simulink model "platoon_blocks_hills"  (R2015b)
settings: Solver=VariableStepAuto  StartTime=0.0  StopTime=50.0  MaxStep=0.001  RelTol=1e-3
undefined symbols (not defined in the file or in its folder): ca1_2, ca1_3, ca1_4, ca1_5, ca1_6, caf1_3, caf1_4, caf1_5, caf1_6, cv1_2, cv1_3, cv1_4, cv1_5, cv1_6, cvf1_3, cvf1_4, cvf1_5, cvf1_6, cx1_2, cx1_3, cx1_4, cx1_5, cx1_6, theta_hill, x_hill
settings Model: Creator=cf5eg  LastModifiedBy=cf5eg

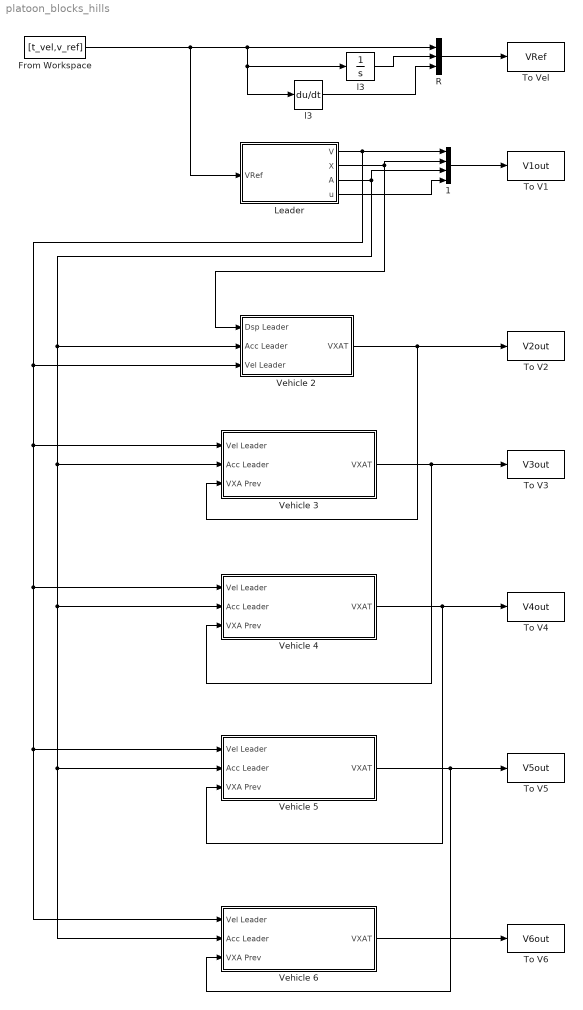
== system platoon_blocks_hills ==
  " 1" : Concatenate  NumInputs=4
  " R" : Concatenate  NumInputs=3
  " l3" : Derivative
  From Workspace : FromWorkspace  VariableName=[t_vel,v_ref]  SampleTime=0
  Leader : Subsystem
  To V1 : ToWorkspace  VariableName=V1out  SaveFormat=Timeseries  SampleTime=-1
  To V2 : ToWorkspace  VariableName=V2out  SaveFormat=Timeseries  SampleTime=-1
  To V3 : ToWorkspace  VariableName=V3out  SaveFormat=Timeseries  SampleTime=-1
  To V4 : ToWorkspace  VariableName=V4out  SaveFormat=Timeseries  SampleTime=-1
  To V5 : ToWorkspace  VariableName=V5out  SaveFormat=Timeseries  SampleTime=-1
  To V6 : ToWorkspace  VariableName=V6out  SaveFormat=Timeseries  SampleTime=-1
  To Vel : ToWorkspace  VariableName=VRef  SaveFormat=Timeseries  SampleTime=-1
  Vehicle 2 : Subsystem
  Vehicle 3 : Subsystem
  Vehicle 4 : Subsystem
  Vehicle 5 : Subsystem
      mask Display: image('car.jpg')
  Vehicle 6 : Subsystem
      mask Display: image('car.jpg')
  l3 : Integrator
  wires:
  " 1"/1 -> To V1/1
  Vehicle 3/1(VXAT) -> Vehicle 4/3(VXA Prev), To V3/1
  l3/1 -> " R"/2
  " l3"/1 -> " R"/3
  " R"/1 -> To Vel/1
  From Workspace/1 -> Leader/1(VRef), " l3"/1, l3/1, " R"/1
  Vehicle 4/1(VXAT) -> Vehicle 5/3(VXA Prev), To V4/1
  Vehicle 5/1(VXAT) -> Vehicle 6/3(VXA Prev), To V5/1
  Leader/2(X) -> Vehicle 2/1(Dsp Leader), " 1"/2
  Leader/3(A) -> " 1"/3, Vehicle 2/2(Acc Leader), Vehicle 6/2(Acc Leader), Vehicle 5/2(Acc Leader), Vehicle 4/2(Acc Leader), Vehicle 3/2(Acc Leader)
  Leader/1(V) -> " 1"/1, Vehicle 2/3(Vel Leader), Vehicle 6/1(Vel Leader), Vehicle 5/1(Vel Leader), Vehicle 4/1(Vel Leader), Vehicle 3/1(Vel Leader)
  Vehicle 6/1(VXAT) -> To V6/1
  Vehicle 2/1(VXAT) -> Vehicle 3/3(VXA Prev), To V2/1
  Leader/4(u) -> " 1"/4

== system platoon_blocks_hills/Leader ==
  VRef : Inport
  " l" : Derivative
  Der Error : Derivative
  Int Error : Integrator
  Sum5 : Sum  Inputs=+++
  Sum7 : Sum  Inputs=|+-
  Transport Delay : TransportDelay  DelayTime=0.1
  Vehicle 1 : Subsystem
  kd : Gain  Gain=0
  ki : Gain  Gain=0.1
  kp : Gain  Gain=0.5
  l : Integrator
  V : Outport
  X : Outport  Port=2
  A : Outport  Port=3
  u : Outport  Port=4
  wires:
  VRef/1 -> Sum7/1
  Sum5/1 -> Transport Delay/1
  Vehicle 1/1(v) -> l/1, Sum7/2, " l"/1, V/1
  Sum7/1 -> Der Error/1, Int Error/1, kp/1
  kp/1 -> Sum5/1
  ki/1 -> Sum5/2
  Int Error/1 -> ki/1
  kd/1 -> Sum5/3
  Der Error/1 -> kd/1
  l/1 -> X/1
  " l"/1 -> A/1
  Transport Delay/1 -> Vehicle 1/1(u)
  Vehicle 1/2(throttle) -> u/1

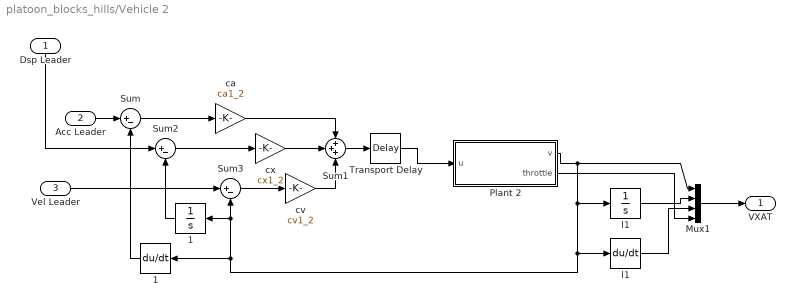
== system platoon_blocks_hills/Vehicle 2 ==
  Dsp Leader : Inport
  Acc Leader : Inport  Port=2
  Vel Leader : Inport  Port=3
  " l1" : Derivative
  1 : Integrator
  "1 " : Derivative
  Mux1 : Mux
  Plant 2 : Subsystem
  Sum : Sum  Inputs=|+-
  Sum1 : Sum  Inputs=+++
  Sum2 : Sum  Inputs=|+-
  Sum3 : Sum  Inputs=|+-
  Transport Delay : TransportDelay  DelayTime=0.1
  ca : Gain  Gain=ca1_2
  cv : Gain  Gain=cv1_2
  cx : Gain  Gain=cx1_2
  l1 : Integrator
  VXAT : Outport
  wires:
  Vel Leader/1 -> Sum3/1
  ca/1 -> Sum1/1
  Sum2/1 -> cx/1
  cx/1 -> Sum1/2
  cv/1 -> Sum1/3
  Sum/1 -> ca/1
  1/1 -> Sum2/2
  "1 "/1 -> Sum/2
  Sum3/1 -> cv/1
  Sum1/1 -> Transport Delay/1
  Plant 2/1(v) -> Mux1/1, l1/1, " l1"/1, Sum3/2, 1/1, "1 "/1
  " l1"/1 -> Mux1/3
  l1/1 -> Mux1/2
  Dsp Leader/1 -> Sum2/1
  Acc Leader/1 -> Sum/1
  Mux1/1 -> VXAT/1
  Transport Delay/1 -> Plant 2/1(u)
  Plant 2/2(throttle) -> Mux1/4

== system platoon_blocks_hills/Vehicle 3 ==
  Vel Leader : Inport
  Acc Leader : Inport  Port=2
  VXA Prev : Inport  Port=3
  Controller 3 : Subsystem
  Demux : Demux
  Mux1 : Mux
  Plant 3 : Subsystem
  Terminator : Terminator
  Transport Delay : TransportDelay  DelayTime=0.1
  VXAT : Outport
  wires:
  Controller 3/1(u) -> Transport Delay/1
  Plant 3/1(v) -> Mux1/1, Controller 3/6(vself)
  Plant 3/2(x) -> Mux1/2
  Plant 3/3(a) -> Mux1/3
  Vel Leader/1 -> Controller 3/2(vl)
  Acc Leader/1 -> Controller 3/1(al)
  VXA Prev/1 -> Demux/1
  Demux/1 -> Controller 3/5(v0)
  Demux/2 -> Controller 3/4(x0)
  Demux/3 -> Controller 3/3(a0)
  Mux1/1 -> VXAT/1
  Transport Delay/1 -> Plant 3/1(u)
  Demux/4 -> Terminator/1
  Plant 3/4(t) -> Mux1/4

== system platoon_blocks_hills/Vehicle 4 ==
  Vel Leader : Inport
  Acc Leader : Inport  Port=2
  VXA Prev : Inport  Port=3
  Controller 4 : Subsystem
  Demux : Demux
  Mux1 : Mux
  Plant 4 : Subsystem
  Terminator : Terminator
  Transport Delay : TransportDelay  DelayTime=0.1
  VXAT : Outport
  wires:
  Controller 4/1(u) -> Transport Delay/1
  Plant 4/1(v) -> Controller 4/6(vself), Mux1/1
  Plant 4/2(x) -> Mux1/2
  Plant 4/3(a) -> Mux1/3
  Vel Leader/1 -> Controller 4/2(vl)
  Acc Leader/1 -> Controller 4/1(al)
  VXA Prev/1 -> Demux/1
  Demux/1 -> Controller 4/5(v0)
  Demux/2 -> Controller 4/4(x0)
  Demux/3 -> Controller 4/3(a0)
  Mux1/1 -> VXAT/1
  Transport Delay/1 -> Plant 4/1(u)
  Demux/4 -> Terminator/1
  Plant 4/4(t) -> Mux1/4

== system platoon_blocks_hills/Vehicle 5 ==
  Vel Leader : Inport
  Acc Leader : Inport  Port=2
  VXA Prev : Inport  Port=3
  Controller 5 : Subsystem
  Demux : Demux
  Mux1 : Mux
  Plant 5 : Subsystem
  Terminator : Terminator
  Transport Delay : TransportDelay  DelayTime=0.1
  VXAT : Outport
  wires:
  Controller 5/1(u) -> Transport Delay/1
  Plant 5/1(v) -> Controller 5/6(vself), Mux1/1
  Plant 5/2(x) -> Mux1/2
  Plant 5/3(a) -> Mux1/3
  Vel Leader/1 -> Controller 5/2(vl)
  Acc Leader/1 -> Controller 5/1(al)
  VXA Prev/1 -> Demux/1
  Demux/1 -> Controller 5/5(v0)
  Demux/2 -> Controller 5/4(x0)
  Demux/3 -> Controller 5/3(a0)
  Mux1/1 -> VXAT/1
  Transport Delay/1 -> Plant 5/1(u)
  Demux/4 -> Terminator/1
  Plant 5/4(t) -> Mux1/4

== system platoon_blocks_hills/Vehicle 6 ==
  Vel Leader : Inport
  Acc Leader : Inport  Port=2
  VXA Prev : Inport  Port=3
  Controller 6 : Subsystem
  Demux : Demux
  Mux1 : Mux
  Plant 6 : Subsystem
  Terminator : Terminator
  Transport Delay : TransportDelay  DelayTime=0.1
  VXAT : Outport
  wires:
  Controller 6/1(u) -> Transport Delay/1
  Plant 6/1(v) -> Controller 6/6(vself), Mux1/1
  Plant 6/2(x) -> Mux1/2
  Plant 6/3(a) -> Mux1/3
  Acc Leader/1 -> Controller 6/1(al)
  VXA Prev/1 -> Demux/1
  Mux1/1 -> VXAT/1
  Transport Delay/1 -> Plant 6/1(u)
  Demux/3 -> Controller 6/3(a0)
  Demux/2 -> Controller 6/4(x0)
  Demux/1 -> Controller 6/5(v0)
  Vel Leader/1 -> Controller 6/2(vl)
  Demux/4 -> Terminator/1
  Plant 6/4(t) -> Mux1/4

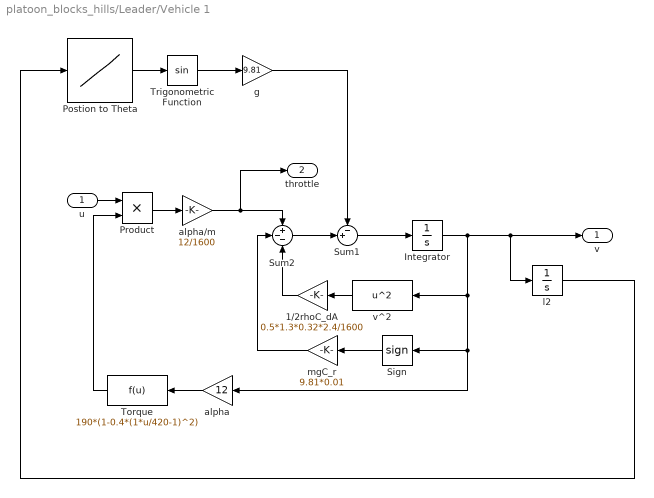
== system platoon_blocks_hills/Leader/Vehicle 1 ==
  u : Inport
  1/2rhoC_dA : Gain  Gain=0.5*1.3*0.32*2.4/1600
  Integrator : Integrator
  Postion to Theta : Lookup_n-D  NumberOfTableDimensions=1  BreakpointsForDimension1=x_hill  Table=theta_hill  InternalRulePriority=Speed  RndMeth=Simplest  InputSameDT=on
  Product : Product
  Sign : Signum  ZeroCross=off
  Sum1 : Sum  Inputs=-+|
  Sum2 : Sum  Inputs=+--
  Torque : Fcn  Expr=190*(1-0.4*(1*u/420-1)^2)
  Trigonometric Function : Trigonometry
  alpha : Gain  Gain=12
  alpha/m : Gain  Gain=12/1600
  g : Gain  Gain=9.81
  l2 : Integrator
  "mgC_r " : Gain  Gain=9.81*0.01
  v^2 : Fcn  Expr=u^2
  v : Outport
  throttle : Outport  Port=2
  wires:
  Product/1 -> alpha/m/1
  alpha/m/1 -> throttle/1, Sum2/1
  alpha/1 -> Torque/1
  Torque/1 -> Product/2
  v^2/1 -> 1/2rhoC_dA/1
  1/2rhoC_dA/1 -> Sum2/3
  Integrator/1 -> l2/1, v/1, Sign/1, alpha/1, v^2/1
  Sum2/1 -> Sum1/2
  "mgC_r "/1 -> Sum2/2
  Sign/1 -> "mgC_r "/1
  u/1 -> Product/1
  l2/1 -> Postion to Theta/1
  Postion to Theta/1 -> Trigonometric Function/1
  Trigonometric Function/1 -> g/1
  Sum1/1 -> Integrator/1
  g/1 -> Sum1/1

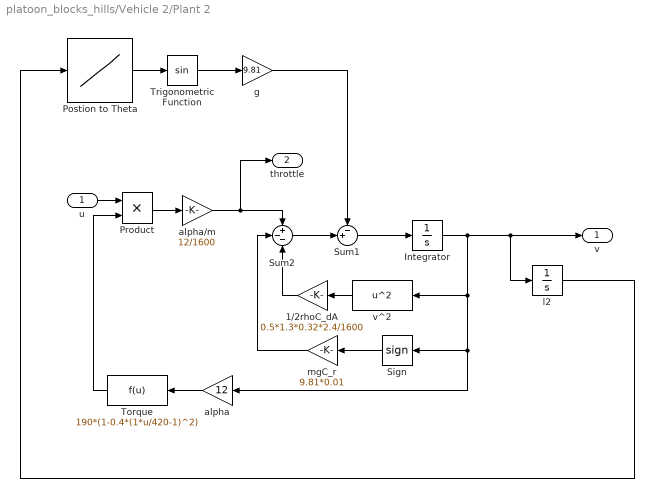
== system platoon_blocks_hills/Vehicle 2/Plant 2 ==
  u : Inport
  1/2rhoC_dA : Gain  Gain=0.5*1.3*0.32*2.4/1600
  Integrator : Integrator
  Postion to Theta : Lookup_n-D  NumberOfTableDimensions=1  BreakpointsForDimension1=x_hill  Table=theta_hill  InternalRulePriority=Speed  RndMeth=Simplest  InputSameDT=on
  Product : Product
  Sign : Signum  ZeroCross=off
  Sum1 : Sum  Inputs=-+|
  Sum2 : Sum  Inputs=+--
  Torque : Fcn  Expr=190*(1-0.4*(1*u/420-1)^2)
  Trigonometric Function : Trigonometry
  alpha : Gain  Gain=12
  alpha/m : Gain  Gain=12/1600
  g : Gain  Gain=9.81
  l2 : Integrator
  "mgC_r " : Gain  Gain=9.81*0.01
  v^2 : Fcn  Expr=u^2
  v : Outport
  throttle : Outport  Port=2
  wires:
  Product/1 -> alpha/m/1
  alpha/m/1 -> throttle/1, Sum2/1
  alpha/1 -> Torque/1
  Torque/1 -> Product/2
  v^2/1 -> 1/2rhoC_dA/1
  1/2rhoC_dA/1 -> Sum2/3
  Integrator/1 -> l2/1, v/1, Sign/1, alpha/1, v^2/1
  Sum2/1 -> Sum1/2
  "mgC_r "/1 -> Sum2/2
  Sign/1 -> "mgC_r "/1
  u/1 -> Product/1
  l2/1 -> Postion to Theta/1
  Postion to Theta/1 -> Trigonometric Function/1
  Trigonometric Function/1 -> g/1
  Sum1/1 -> Integrator/1
  g/1 -> Sum1/1

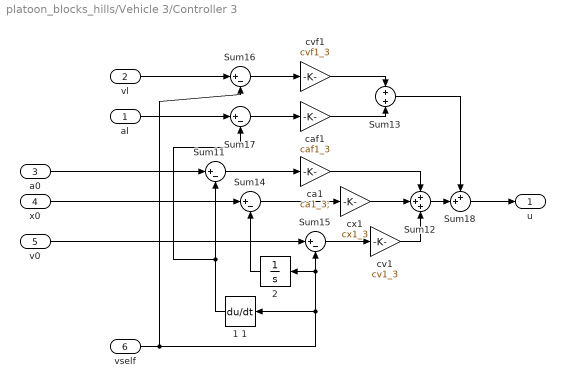
== system platoon_blocks_hills/Vehicle 3/Controller 3 ==
  al : Inport
  vl : Inport  Port=2
  a0 : Inport  Port=3
  x0 : Inport  Port=4
  v0 : Inport  Port=5
  vself : Inport  Port=6
  1 1 : Derivative
  2 : Integrator
  Sum{11,14..17} (5 alike) : Sum  Inputs=|+-
  Sum12 : Sum  Inputs=+++
  Sum13 : Sum  Inputs=+|+
  Sum18 : Sum  Inputs=++|
  ca1 : Gain  Gain=ca1_3;
  caf1 : Gain  Gain=caf1_3
  cv1 : Gain  Gain=cv1_3
  cvf1 : Gain  Gain=cvf1_3
  cx1 : Gain  Gain=cx1_3
  u : Outport
  wires:
  vl/1 -> Sum16/1
  ca1/1 -> Sum12/1
  Sum18/1 -> u/1
  Sum14/1 -> cx1/1
  cx1/1 -> Sum12/2
  cv1/1 -> Sum12/3
  Sum11/1 -> ca1/1
  2/1 -> Sum14/2
  1 1/1 -> Sum17/2, Sum11/2
  Sum15/1 -> cv1/1
  Sum16/1 -> cvf1/1
  Sum17/1 -> caf1/1
  caf1/1 -> Sum13/2
  cvf1/1 -> Sum13/1
  Sum12/1 -> Sum18/2
  Sum13/1 -> Sum18/1
  vself/1 -> Sum16/2, Sum15/2, 2/1, 1 1/1
  al/1 -> Sum17/1
  a0/1 -> Sum11/1
  v0/1 -> Sum15/1
  x0/1 -> Sum14/1

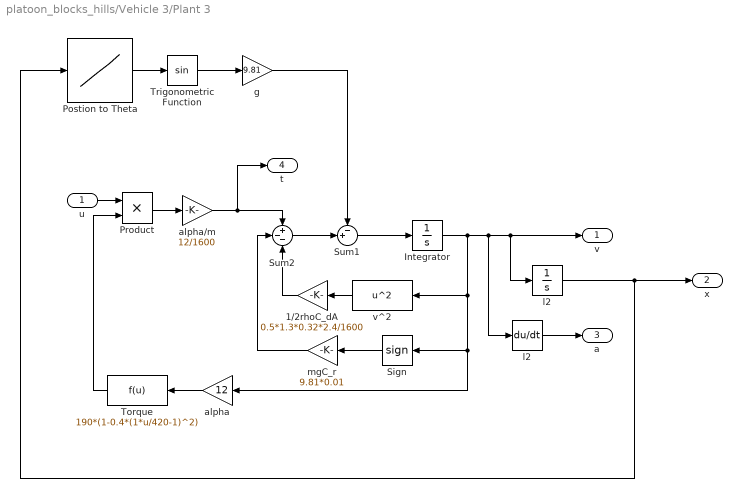
== system platoon_blocks_hills/Vehicle 3/Plant 3 ==
  u : Inport
  " l2" : Derivative
  1/2rhoC_dA : Gain  Gain=0.5*1.3*0.32*2.4/1600
  Integrator : Integrator
  Postion to Theta : Lookup_n-D  NumberOfTableDimensions=1  BreakpointsForDimension1=x_hill  Table=theta_hill  InternalRulePriority=Speed  RndMeth=Simplest  InputSameDT=on
  Product : Product
  Sign : Signum  ZeroCross=off
  Sum1 : Sum  Inputs=-+|
  Sum2 : Sum  Inputs=+--
  Torque : Fcn  Expr=190*(1-0.4*(1*u/420-1)^2)
  Trigonometric Function : Trigonometry
  alpha : Gain  Gain=12
  alpha/m : Gain  Gain=12/1600
  g : Gain  Gain=9.81
  l2 : Integrator
  "mgC_r " : Gain  Gain=9.81*0.01
  v^2 : Fcn  Expr=u^2
  v : Outport
  x : Outport  Port=2
  a : Outport  Port=3
  t : Outport  Port=4
  wires:
  Product/1 -> alpha/m/1
  alpha/m/1 -> t/1, Sum2/1
  alpha/1 -> Torque/1
  Torque/1 -> Product/2
  v^2/1 -> 1/2rhoC_dA/1
  1/2rhoC_dA/1 -> Sum2/3
  Integrator/1 -> " l2"/1, l2/1, v/1, Sign/1, alpha/1, v^2/1
  Sum2/1 -> Sum1/2
  "mgC_r "/1 -> Sum2/2
  Sign/1 -> "mgC_r "/1
  u/1 -> Product/1
  " l2"/1 -> a/1
  l2/1 -> x/1, Postion to Theta/1
  Postion to Theta/1 -> Trigonometric Function/1
  Trigonometric Function/1 -> g/1
  Sum1/1 -> Integrator/1
  g/1 -> Sum1/1

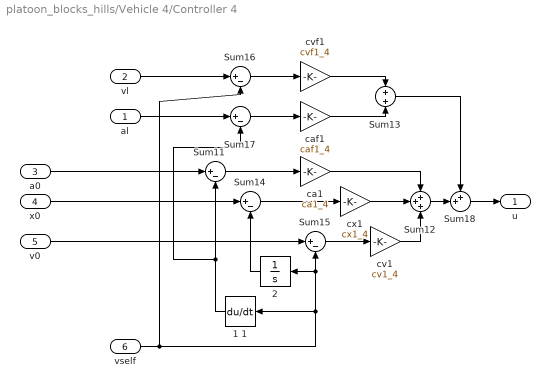
== system platoon_blocks_hills/Vehicle 4/Controller 4 ==
  al : Inport
  vl : Inport  Port=2
  a0 : Inport  Port=3
  x0 : Inport  Port=4
  v0 : Inport  Port=5
  vself : Inport  Port=6
  1 1 : Derivative
  2 : Integrator
  Sum{11,14..17} (5 alike) : Sum  Inputs=|+-
  Sum12 : Sum  Inputs=+++
  Sum13 : Sum  Inputs=+|+
  Sum18 : Sum  Inputs=++|
  ca1 : Gain  Gain=ca1_4
  caf1 : Gain  Gain=caf1_4
  cv1 : Gain  Gain=cv1_4
  cvf1 : Gain  Gain=cvf1_4
  cx1 : Gain  Gain=cx1_4
  u : Outport
  wires:
  vl/1 -> Sum16/1
  ca1/1 -> Sum12/1
  Sum18/1 -> u/1
  Sum14/1 -> cx1/1
  cx1/1 -> Sum12/2
  cv1/1 -> Sum12/3
  Sum11/1 -> ca1/1
  2/1 -> Sum14/2
  1 1/1 -> Sum17/2, Sum11/2
  Sum15/1 -> cv1/1
  Sum16/1 -> cvf1/1
  Sum17/1 -> caf1/1
  caf1/1 -> Sum13/2
  cvf1/1 -> Sum13/1
  Sum12/1 -> Sum18/2
  Sum13/1 -> Sum18/1
  vself/1 -> Sum16/2, Sum15/2, 2/1, 1 1/1
  al/1 -> Sum17/1
  a0/1 -> Sum11/1
  v0/1 -> Sum15/1
  x0/1 -> Sum14/1

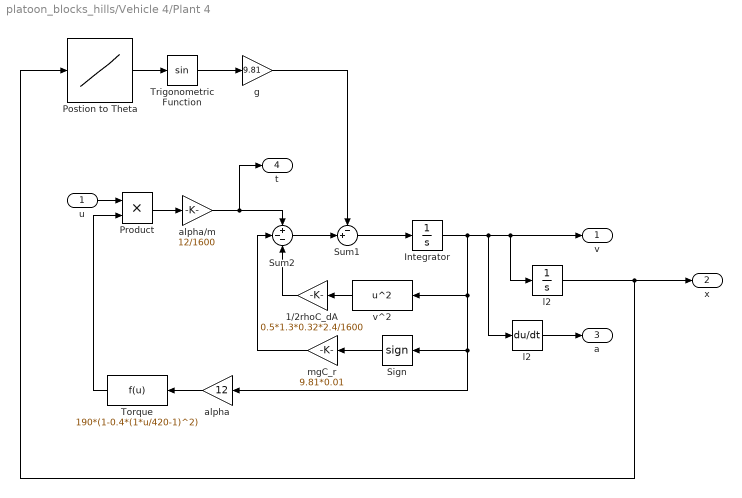
== system platoon_blocks_hills/Vehicle 4/Plant 4 ==
  u : Inport
  " l2" : Derivative
  1/2rhoC_dA : Gain  Gain=0.5*1.3*0.32*2.4/1600
  Integrator : Integrator
  Postion to Theta : Lookup_n-D  NumberOfTableDimensions=1  BreakpointsForDimension1=x_hill  Table=theta_hill  InternalRulePriority=Speed  RndMeth=Simplest  InputSameDT=on
  Product : Product
  Sign : Signum  ZeroCross=off
  Sum1 : Sum  Inputs=-+|
  Sum2 : Sum  Inputs=+--
  Torque : Fcn  Expr=190*(1-0.4*(1*u/420-1)^2)
  Trigonometric Function : Trigonometry
  alpha : Gain  Gain=12
  alpha/m : Gain  Gain=12/1600
  g : Gain  Gain=9.81
  l2 : Integrator
  "mgC_r " : Gain  Gain=9.81*0.01
  v^2 : Fcn  Expr=u^2
  v : Outport
  x : Outport  Port=2
  a : Outport  Port=3
  t : Outport  Port=4
  wires:
  Product/1 -> alpha/m/1
  alpha/m/1 -> t/1, Sum2/1
  alpha/1 -> Torque/1
  Torque/1 -> Product/2
  v^2/1 -> 1/2rhoC_dA/1
  1/2rhoC_dA/1 -> Sum2/3
  Integrator/1 -> " l2"/1, l2/1, v/1, Sign/1, alpha/1, v^2/1
  Sum2/1 -> Sum1/2
  "mgC_r "/1 -> Sum2/2
  Sign/1 -> "mgC_r "/1
  u/1 -> Product/1
  " l2"/1 -> a/1
  l2/1 -> x/1, Postion to Theta/1
  Postion to Theta/1 -> Trigonometric Function/1
  Trigonometric Function/1 -> g/1
  Sum1/1 -> Integrator/1
  g/1 -> Sum1/1

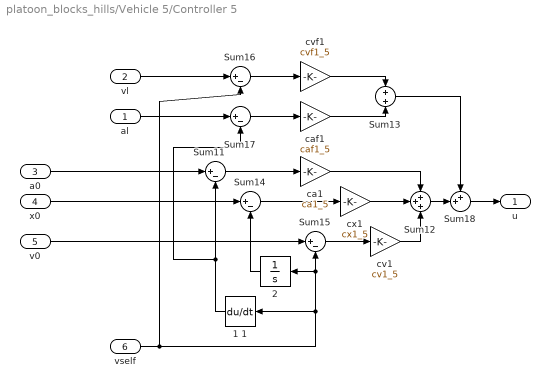
== system platoon_blocks_hills/Vehicle 5/Controller 5 ==
  al : Inport
  vl : Inport  Port=2
  a0 : Inport  Port=3
  x0 : Inport  Port=4
  v0 : Inport  Port=5
  vself : Inport  Port=6
  1 1 : Derivative
  2 : Integrator
  Sum{11,14..17} (5 alike) : Sum  Inputs=|+-
  Sum12 : Sum  Inputs=+++
  Sum13 : Sum  Inputs=+|+
  Sum18 : Sum  Inputs=++|
  ca1 : Gain  Gain=ca1_5
  caf1 : Gain  Gain=caf1_5
  cv1 : Gain  Gain=cv1_5
  cvf1 : Gain  Gain=cvf1_5
  cx1 : Gain  Gain=cx1_5
  u : Outport
  wires:
  vl/1 -> Sum16/1
  ca1/1 -> Sum12/1
  Sum18/1 -> u/1
  Sum14/1 -> cx1/1
  cx1/1 -> Sum12/2
  cv1/1 -> Sum12/3
  Sum11/1 -> ca1/1
  2/1 -> Sum14/2
  1 1/1 -> Sum17/2, Sum11/2
  Sum15/1 -> cv1/1
  Sum16/1 -> cvf1/1
  Sum17/1 -> caf1/1
  caf1/1 -> Sum13/2
  cvf1/1 -> Sum13/1
  Sum12/1 -> Sum18/2
  Sum13/1 -> Sum18/1
  vself/1 -> Sum16/2, Sum15/2, 2/1, 1 1/1
  al/1 -> Sum17/1
  a0/1 -> Sum11/1
  v0/1 -> Sum15/1
  x0/1 -> Sum14/1

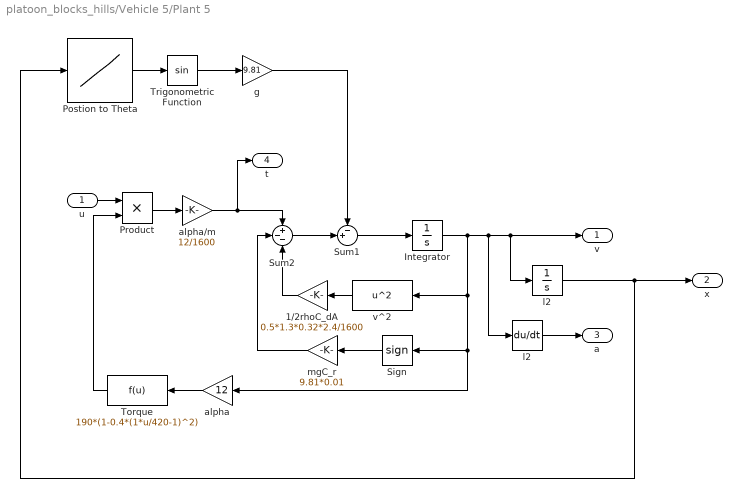
== system platoon_blocks_hills/Vehicle 5/Plant 5 ==
  u : Inport
  " l2" : Derivative
  1/2rhoC_dA : Gain  Gain=0.5*1.3*0.32*2.4/1600
  Integrator : Integrator
  Postion to Theta : Lookup_n-D  NumberOfTableDimensions=1  BreakpointsForDimension1=x_hill  Table=theta_hill  InternalRulePriority=Speed  RndMeth=Simplest  InputSameDT=on
  Product : Product
  Sign : Signum  ZeroCross=off
  Sum1 : Sum  Inputs=-+|
  Sum2 : Sum  Inputs=+--
  Torque : Fcn  Expr=190*(1-0.4*(1*u/420-1)^2)
  Trigonometric Function : Trigonometry
  alpha : Gain  Gain=12
  alpha/m : Gain  Gain=12/1600
  g : Gain  Gain=9.81
  l2 : Integrator
  "mgC_r " : Gain  Gain=9.81*0.01
  v^2 : Fcn  Expr=u^2
  v : Outport
  x : Outport  Port=2
  a : Outport  Port=3
  t : Outport  Port=4
  wires:
  Product/1 -> alpha/m/1
  alpha/m/1 -> t/1, Sum2/1
  alpha/1 -> Torque/1
  Torque/1 -> Product/2
  v^2/1 -> 1/2rhoC_dA/1
  1/2rhoC_dA/1 -> Sum2/3
  Integrator/1 -> " l2"/1, l2/1, v/1, Sign/1, alpha/1, v^2/1
  Sum2/1 -> Sum1/2
  "mgC_r "/1 -> Sum2/2
  Sign/1 -> "mgC_r "/1
  u/1 -> Product/1
  " l2"/1 -> a/1
  l2/1 -> x/1, Postion to Theta/1
  Postion to Theta/1 -> Trigonometric Function/1
  Trigonometric Function/1 -> g/1
  Sum1/1 -> Integrator/1
  g/1 -> Sum1/1

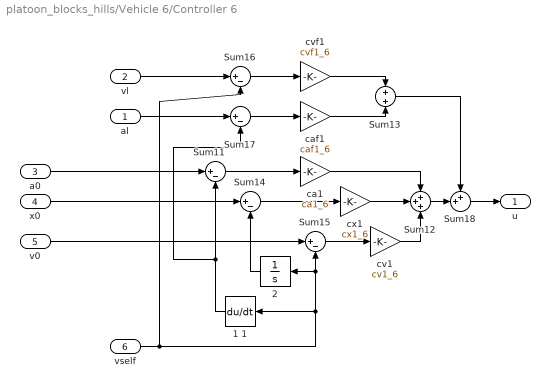
== system platoon_blocks_hills/Vehicle 6/Controller 6 ==
  al : Inport
  vl : Inport  Port=2
  a0 : Inport  Port=3
  x0 : Inport  Port=4
  v0 : Inport  Port=5
  vself : Inport  Port=6
  1 1 : Derivative
  2 : Integrator
  Sum{11,14..17} (5 alike) : Sum  Inputs=|+-
  Sum12 : Sum  Inputs=+++
  Sum13 : Sum  Inputs=+|+
  Sum18 : Sum  Inputs=++|
  ca1 : Gain  Gain=ca1_6
  caf1 : Gain  Gain=caf1_6
  cv1 : Gain  Gain=cv1_6
  cvf1 : Gain  Gain=cvf1_6
  cx1 : Gain  Gain=cx1_6
  u : Outport
  wires:
  vl/1 -> Sum16/1
  ca1/1 -> Sum12/1
  Sum18/1 -> u/1
  Sum14/1 -> cx1/1
  cx1/1 -> Sum12/2
  cv1/1 -> Sum12/3
  Sum11/1 -> ca1/1
  2/1 -> Sum14/2
  1 1/1 -> Sum17/2, Sum11/2
  Sum15/1 -> cv1/1
  Sum16/1 -> cvf1/1
  Sum17/1 -> caf1/1
  caf1/1 -> Sum13/2
  cvf1/1 -> Sum13/1
  Sum12/1 -> Sum18/2
  Sum13/1 -> Sum18/1
  vself/1 -> Sum16/2, Sum15/2, 2/1, 1 1/1
  al/1 -> Sum17/1
  a0/1 -> Sum11/1
  v0/1 -> Sum15/1
  x0/1 -> Sum14/1

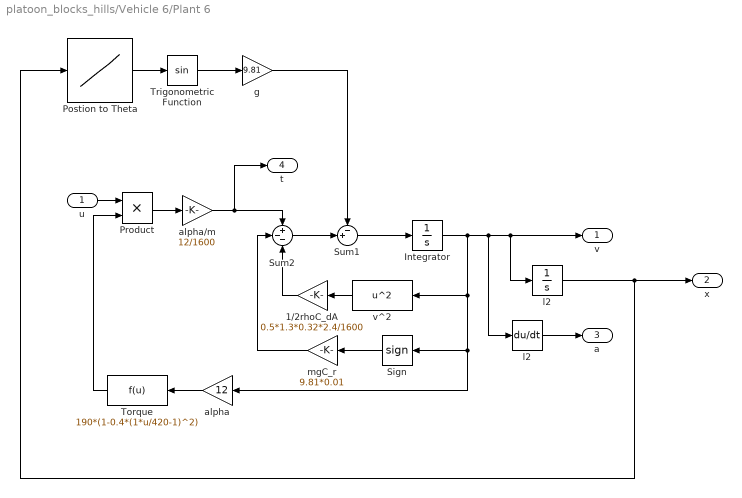
== system platoon_blocks_hills/Vehicle 6/Plant 6 ==
  u : Inport
  " l2" : Derivative
  1/2rhoC_dA : Gain  Gain=0.5*1.3*0.32*2.4/1600
  Integrator : Integrator
  Postion to Theta : Lookup_n-D  NumberOfTableDimensions=1  BreakpointsForDimension1=x_hill  Table=theta_hill  InternalRulePriority=Speed  RndMeth=Simplest  InputSameDT=on
  Product : Product
  Sign : Signum  ZeroCross=off
  Sum1 : Sum  Inputs=-+|
  Sum2 : Sum  Inputs=+--
  Torque : Fcn  Expr=190*(1-0.4*(1*u/420-1)^2)
  Trigonometric Function : Trigonometry
  alpha : Gain  Gain=12
  alpha/m : Gain  Gain=12/1600
  g : Gain  Gain=9.81
  l2 : Integrator
  "mgC_r " : Gain  Gain=9.81*0.01
  v^2 : Fcn  Expr=u^2
  v : Outport
  x : Outport  Port=2
  a : Outport  Port=3
  t : Outport  Port=4
  wires:
  Product/1 -> alpha/m/1
  alpha/m/1 -> t/1, Sum2/1
  alpha/1 -> Torque/1
  Torque/1 -> Product/2
  v^2/1 -> 1/2rhoC_dA/1
  1/2rhoC_dA/1 -> Sum2/3
  Integrator/1 -> " l2"/1, l2/1, v/1, Sign/1, alpha/1, v^2/1
  Sum2/1 -> Sum1/2
  "mgC_r "/1 -> Sum2/2
  Sign/1 -> "mgC_r "/1
  u/1 -> Product/1
  " l2"/1 -> a/1
  l2/1 -> x/1, Postion to Theta/1
  Postion to Theta/1 -> Trigonometric Function/1
  Trigonometric Function/1 -> g/1
  Sum1/1 -> Integrator/1
  g/1 -> Sum1/1
